simulink model "QAM_mixer"  (R2016b)
settings: Solver=FixedStepDiscrete  StartTime=0.0  StopTime=10  RelTol=1e-3
libraries: commdigbbndam3 x16, hdlsllib x5, dspsrcs4 x4, simulink x1, dspxfrm3 x1
settings Model: DataTypeOverride=Off  NumberOfSteps=100  Creator=jake  LastModifiedBy=jake
settings DataIOCC: SaveOutput=off  SaveTime=off
settings OptimizationCC: BlockReduction=off  ConditionallyExecuteInputs=off  DefaultParameterBehavior=Inlined
settings DebuggingCC: AlgebraicLoopMsg=error  SingleTaskRateTransMsg=error  StrictBusMsg=ErrorOnBusTreatedAsVector
settings HardwareCC: ProdBitPerPointer=32  ProdBitPerSizeT=32  ProdBitPerPtrDiffT=32  ProdLargestAtomicFloat=None  ProdIntDivRoundTo=Undefined  ProdEndianess=Unspecified  ProdWordSize=32  ProdHWDeviceType=ASIC/FPGA->ASIC/FPGA  ProdEqTarget=off
settings GRTTargetCC: TargetLangStandard=C89/C90 (ANSI)

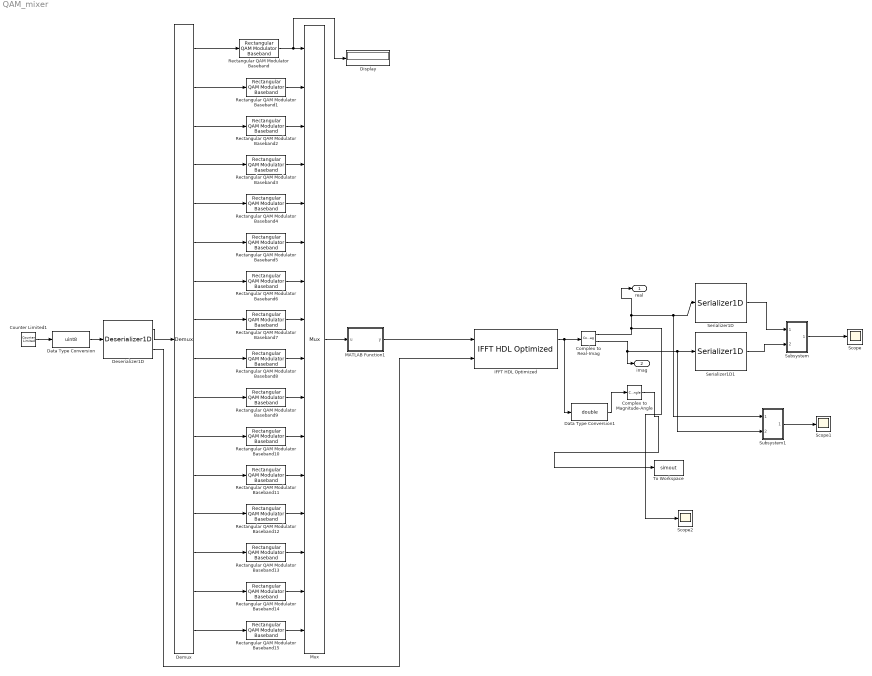
== system QAM_mixer ==
  Complex to Magnitude-Angle : ComplexToMagnitudeAngle  Output=Magnitude
  Complex to Real-Imag : ComplexToRealImag
  Counter Limited1 : simulink/Sources/Counter Limited  uplimit=14  tsamp=-1
  Data Type Conversion : DataTypeConversion  OutDataTypeStr=uint8
  Data Type Conversion1 : DataTypeConversion  OutDataTypeStr=double
  Demux : Demux  Outputs=16
  Deserializer1D : hdlsllib/HDL Operations/Deserializer1D  Ratio=16  IdleCycles=0  InitialCondition=0  startIn=off  validIn=off  validOut=on  inputDataDimensions=-1  inputSampleTime=-1  inputSignalType=auto
  Display : Display
  IFFT HDL Optimized : dspxfrm3/IFFT HDL Optimized  Architecture=Streaming Radix 2^2  ComplexMultiplication=Use 3 multipliers and 5 adders  BitReversedOutput=off  BitReversedInput=on  Normalize=off  FFTLength=16  SimulateUsing=Code generation  RoundingMethod=Floor  ResetInputPort=off  StartOutputPort=off  EndOutputPort=off
  MATLAB Function1 : MATLAB Function  TreatAsAtomicUnit=on
  Mux : Mux  Inputs=16
  Rectangular QAM Modulator Baseband{,1..15} (16 alike) : commdigbbndam3/Rectangular QAM Modulator Baseband  M=16  InType=Integer  Enc=Gray  Mapping=[0:15]  PowType=Min. distance between symbols  MinDist=2  AvgPow=1  PeakPow=1  Ph=0  outDtype=Fixed-point  outWordLen=16  outUDDataType=sfix(16)  outFracLenMode=Best precision  outFracLen=15  outDataTypeStr=fixdt(1,16)  outLastDataTypeStr=fixdt(1,16)
  Scope : Scope
  Scope1 : Scope
  Scope2 : Scope
  Serializer1D : hdlsllib/HDL Operations/Serializer1D  Ratio=16  IdleCycles=0  validIn=off  startOut=off  validOut=off  inputDataDimensions=-1  inputSampleTime=-1  inputSignalType=auto
  Serializer1D1 : hdlsllib/HDL Operations/Serializer1D  Ratio=16  IdleCycles=0  validIn=off  startOut=off  validOut=off  inputDataDimensions=-1  inputSampleTime=-1  inputSignalType=auto
  Subsystem : Subsystem
  Subsystem1 : Subsystem
  To Workspace : ToWorkspace  VariableName=simout  SampleTime=-1
  real : Outport  SignalName=ifft_real
  imag : Outport  Port=2  SignalName=ifft_imag
  wires:
  Demux/1 -> Rectangular QAM Modulator Baseband/1
  Demux/2 -> Rectangular QAM Modulator Baseband1/1
  Demux/3 -> Rectangular QAM Modulator Baseband2/1
  Demux/4 -> Rectangular QAM Modulator Baseband3/1
  Demux/5 -> Rectangular QAM Modulator Baseband4/1
  Demux/6 -> Rectangular QAM Modulator Baseband5/1
  Demux/7 -> Rectangular QAM Modulator Baseband6/1
  Demux/8 -> Rectangular QAM Modulator Baseband7/1
  Demux/9 -> Rectangular QAM Modulator Baseband8/1
  Demux/10 -> Rectangular QAM Modulator Baseband9/1
  Demux/11 -> Rectangular QAM Modulator Baseband10/1
  Demux/12 -> Rectangular QAM Modulator Baseband11/1
  Demux/13 -> Rectangular QAM Modulator Baseband12/1
  Demux/14 -> Rectangular QAM Modulator Baseband13/1
  Demux/15 -> Rectangular QAM Modulator Baseband14/1
  Demux/16 -> Rectangular QAM Modulator Baseband15/1
  Rectangular QAM Modulator Baseband15/1 -> Mux/16
  Rectangular QAM Modulator Baseband14/1 -> Mux/15
  Rectangular QAM Modulator Baseband13/1 -> Mux/14
  Rectangular QAM Modulator Baseband12/1 -> Mux/13
  Rectangular QAM Modulator Baseband11/1 -> Mux/12
  Rectangular QAM Modulator Baseband10/1 -> Mux/11
  Rectangular QAM Modulator Baseband9/1 -> Mux/10
  Rectangular QAM Modulator Baseband8/1 -> Mux/9
  Rectangular QAM Modulator Baseband/1 -> Display/1, Mux/1
  Rectangular QAM Modulator Baseband1/1 -> Mux/2
  Rectangular QAM Modulator Baseband2/1 -> Mux/3
  Rectangular QAM Modulator Baseband3/1 -> Mux/4
  Rectangular QAM Modulator Baseband4/1 -> Mux/5
  Rectangular QAM Modulator Baseband5/1 -> Mux/6
  Rectangular QAM Modulator Baseband6/1 -> Mux/7
  Rectangular QAM Modulator Baseband7/1 -> Mux/8
  Mux/1 -> MATLAB Function1/1(u)
  IFFT HDL Optimized/1 -> Data Type Conversion1/1, Complex to Real-Imag/1
  Complex to Real-Imag/1 -> Scope2/1, Subsystem1/1(Real), Serializer1D/1, real/1
  Deserializer1D/1 -> Demux/1
  Counter Limited1/1 -> Data Type Conversion/1
  Data Type Conversion/1 -> Deserializer1D/1
  Complex to Magnitude-Angle/1 -> To Workspace/1
  Data Type Conversion1/1 -> Complex to Magnitude-Angle/1
  MATLAB Function1/1(y) -> IFFT HDL Optimized/1
  Deserializer1D/2 -> IFFT HDL Optimized/2
  Complex to Real-Imag/2 -> Subsystem1/2(Imag), Serializer1D1/1, imag/1
  Subsystem/1(Baseband Mixed Signal) -> Scope/1
  Serializer1D1/1 -> Subsystem/2(Imag)
  Serializer1D/1 -> Subsystem/1(Real)
  Subsystem1/1(Baseband Mixed Signal) -> Scope1/1

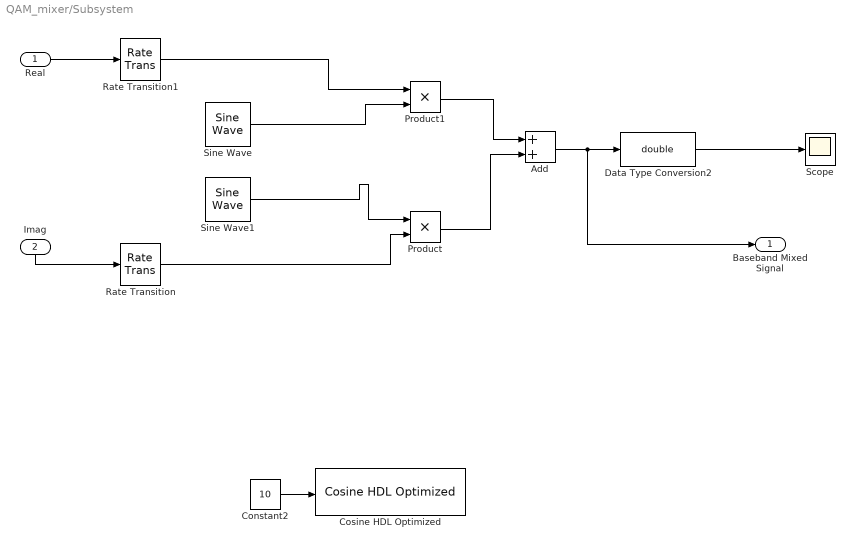
== system QAM_mixer/Subsystem ==
  Real : Inport
  Imag : Inport  Port=2
  Add : Sum
  Constant2 : Constant  Value=10  VectorParams1D=off  OutDataTypeStr=int8
  Cosine HDL Optimized : hdlsllib/Lookup Tables/Cosine HDL Optimized  OutputFormula=sin(2*pi*u) and cos(2*pi*u)  NumDataPoints=64  TableDataTypeStr=fixdt(1,16,0)  SimulateLUTROMDelay=off
  Data Type Conversion2 : DataTypeConversion  OutDataTypeStr=double
  Product : Product
  Product1 : Product
  Rate Transition : RateTransition
  Rate Transition1 : RateTransition
  Scope : Scope
  Sine Wave : dspsrcs4/Sine Wave  Amplitude=1  Frequency=1000  Phase=0  SampleMode=Discrete  OutComplex=Real  CompMethod=Table lookup  TableSize=Speed  SampleTime=1/10000  SamplesPerFrame=1  ResetState=Restart at time zero  OutputFrames=off  dataType=Fixed-point  wordLen=16  udDataType=sfix(16)  fracBitsMode=User-defined  numFracBits=14  OutDataTypeStr=fixdt(1,16,14)  LastOutDataTypeStr=fixdt(1,16,14)
  Sine Wave1 : dspsrcs4/Sine Wave  Amplitude=1  Frequency=1000  Phase=pi/2  SampleMode=Discrete  OutComplex=Real  CompMethod=Table lookup  TableSize=Speed  SampleTime=1/10000  SamplesPerFrame=1  ResetState=Restart at time zero  OutputFrames=off  dataType=Fixed-point  wordLen=16  udDataType=sfix(16)  fracBitsMode=User-defined  numFracBits=14  OutDataTypeStr=fixdt(1,16,14)  LastOutDataTypeStr=fixdt(1,16,14)
  Baseband Mixed Signal : Outport
  wires:
  Data Type Conversion2/1 -> Scope/1
  Rate Transition1/1 -> Product1/1
  Rate Transition/1 -> Product/2
  Product1/1 -> Add/1
  Product/1 -> Add/2
  Add/1 -> Baseband Mixed Signal/1, Data Type Conversion2/1
  Sine Wave/1 -> Product1/2
  Sine Wave1/1 -> Product/1
  Constant2/1 -> Cosine HDL Optimized/1
  Real/1 -> Rate Transition1/1
  Imag/1 -> Rate Transition/1

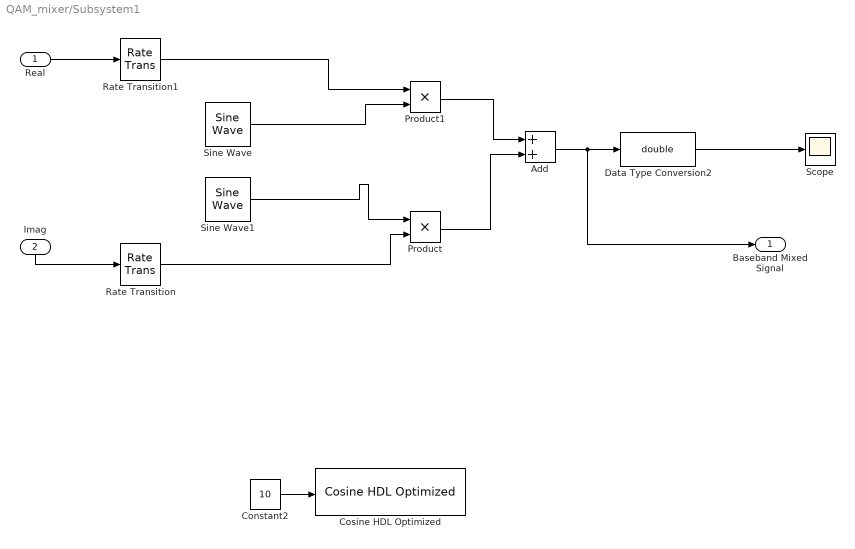
== system QAM_mixer/Subsystem1 ==
  Real : Inport
  Imag : Inport  Port=2
  Add : Sum
  Constant2 : Constant  Value=10  VectorParams1D=off  OutDataTypeStr=int8
  Cosine HDL Optimized : hdlsllib/Lookup Tables/Cosine HDL Optimized  OutputFormula=sin(2*pi*u) and cos(2*pi*u)  NumDataPoints=64  TableDataTypeStr=fixdt(1,16,0)  SimulateLUTROMDelay=off
  Data Type Conversion2 : DataTypeConversion  OutDataTypeStr=double
  Product : Product
  Product1 : Product
  Rate Transition : RateTransition
  Rate Transition1 : RateTransition
  Scope : Scope
  Sine Wave : dspsrcs4/Sine Wave  Amplitude=1  Frequency=10  Phase=0  SampleMode=Discrete  OutComplex=Real  CompMethod=Table lookup  TableSize=Speed  SampleTime=1/1000  SamplesPerFrame=1  ResetState=Restart at time zero  OutputFrames=off  dataType=Fixed-point  wordLen=16  udDataType=sfix(16)  fracBitsMode=User-defined  numFracBits=14  OutDataTypeStr=fixdt(1,16,14)  LastOutDataTypeStr=fixdt(1,16,14)
  Sine Wave1 : dspsrcs4/Sine Wave  Amplitude=1  Frequency=10  Phase=pi/2  SampleMode=Discrete  OutComplex=Real  CompMethod=Table lookup  TableSize=Speed  SampleTime=1/1000  SamplesPerFrame=1  ResetState=Restart at time zero  OutputFrames=off  dataType=Fixed-point  wordLen=16  udDataType=sfix(16)  fracBitsMode=User-defined  numFracBits=14  OutDataTypeStr=fixdt(1,16,14)  LastOutDataTypeStr=fixdt(1,16,14)
  Baseband Mixed Signal : Outport
  wires:
  Data Type Conversion2/1 -> Scope/1
  Rate Transition1/1 -> Product1/1
  Rate Transition/1 -> Product/2
  Product1/1 -> Add/1
  Product/1 -> Add/2
  Add/1 -> Baseband Mixed Signal/1, Data Type Conversion2/1
  Sine Wave/1 -> Product1/2
  Sine Wave1/1 -> Product/1
  Constant2/1 -> Cosine HDL Optimized/1
  Real/1 -> Rate Transition1/1
  Imag/1 -> Rate Transition/1

== matlab function QAM_mixer/MATLAB Function1 ==
  data: u input; y output
function y = bit_reverse(u)
    coder.varsize('bit-reverse', [1024 1]);
    u = bitrevorder(u);
y = u;
end
